simulink model "rovertest"  (R2023a)
settings: Solver=VariableStepAuto  StartTime=0.0  StopTime=60  RelTol=1e-3
libraries: robotalgslib x1
settings Model: Creator=ockap  LastModifiedBy=ockap

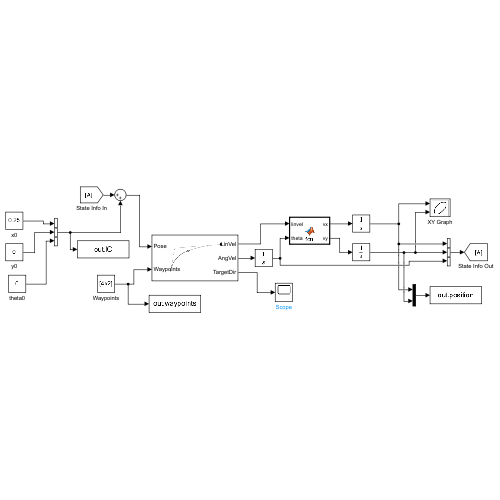
[thumbnail: Simulink's stored preview of the top-level diagram]
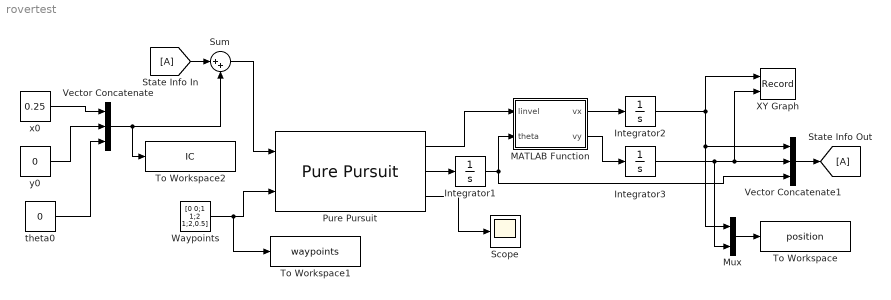
== system rovertest ==
  Integrator1 : Integrator
  Integrator2 : Integrator
  Integrator3 : Integrator
  MATLAB Function : MATLAB Function  TreatAsAtomicUnit=on
  Mux : Mux  Inputs=2
  Pure Pursuit : robotalgslib/Pure Pursuit  DesiredLinearVelocity=0.05  MaxAngularVelocity=1.0  LookaheadDistance=0.2  TargetDirPort=on  SimulateUsing=Code generation
      settings: LibrarySourceBlock=robotmobilelib/Pure Pursuit
  Scope : Scope
  State Info In : From
  State Info Out : Goto
  Sum : Sum  Inputs=|++
  To Workspace : ToWorkspace  VariableName=position  SaveFormat=Timeseries  SampleTime=-1
  To Workspace1 : ToWorkspace  VariableName=waypoints  SampleTime=-1
      settings: Save2DSignal=2-D array (concatenate along first dimension)
  To Workspace2 : ToWorkspace  VariableName=IC  SampleTime=-1
      settings: Save2DSignal=2-D array (concatenate along first dimension)
  Vector Concatenate : Concatenate  NumInputs=3
  Vector Concatenate1 : Concatenate  NumInputs=3
  Waypoints : Constant  Value=[0 0;1 1;2 1;2,0.5]  VectorParams1D=off
  XY Graph : Record  FileSettingsInternal="{\"entries\":[{\"content\":{\"excelSettings\":{\"content\":{},\"type\":\"Streamout.ExcelSettings\"}},\"type\":\"Streamout.FileSettingStorage\",\"uuid\":\"\"}],\"packageUris\":[\"http:\\/\\/schema.mathworks.com\\/mf0\\/streamout_blocks\\/R2020a\"],\"version\":\"1.0\"}"  Layout=[1 1]  SignalsInternal="{\"entries\":[{\"content\":{\"signals\":[{\"content\":{\"blockPath\":[],\"dimensions\":[1],\"domain\":\"\",\"lineColor\":\"#a2142f\",\"plots\":[1],\"port\":1,\"sid\":[\"\"],\"signalID\":19,\"signalName\":\"Integrator2\"},\"type\":\"RecordBlkView.Signal\",\"uuid\":\"\"},{\"content\":{\"blockPath\":[],\"dimensions\":[1],\"domain\":\"\",\"lineColor\":\"#139fff\",\"plots\":[1],\"port\":2,\"sid\":[\"\"],\"signalID\":23,\"signalName\":\"Integrator3\"},\"type\":\"RecordBlkView.Signal\",\"uuid\":\"\"}]},\"type\":\"RecordBlkView.InputSignals\",\"uuid\":\"\"}],\"packageUris\":[\"http:\\/\\/schema.mathworks.com\\/mf0\\/streamout_blocks\\/R2020a\"],\"version\":\"1.0\"}"  VisualizationBindings="{\"xyplotplugin\":{\"info\":[{\"series\":[{\"bindingParametersList\":[{\"parameter\":\"X-Axis\",\"signalID\":19,\"signalName\":\"Integrator2\"},{\"parameter\":\"Y-Axis\",\"signalID\":23,\"signalName\":\"Integrator3\"}],\"seriesID\":3777}],\"subplotID\":1}]}}"  CompatibilityTag=XY
  theta0 : Constant  Value=0
  x0 : Constant  Value=0.25
  y0 : Constant  Value=0
  wires:
  Pure Pursuit/2 -> Integrator1/1
  Pure Pursuit/3 -> Scope/1
  State Info In/1 -> Sum/1
  Pure Pursuit/1 -> MATLAB Function/1(linvel)
  Integrator1/1 -> Vector Concatenate1/3, MATLAB Function/2(theta)
  MATLAB Function/1(vx) -> Integrator2/1
  MATLAB Function/2(vy) -> Integrator3/1
  Integrator2/1 -> Mux/1, Vector Concatenate1/1, XY Graph/1
  Vector Concatenate1/1 -> State Info Out/1
  Sum/1 -> Pure Pursuit/1
  Vector Concatenate/1 -> To Workspace2/1, Sum/2
  x0/1 -> Vector Concatenate/1
  y0/1 -> Vector Concatenate/2
  theta0/1 -> Vector Concatenate/3
  Waypoints/1 -> To Workspace1/1, Pure Pursuit/2
  Integrator3/1 -> Vector Concatenate1/2, XY Graph/2, Mux/2
  Mux/1 -> To Workspace/1

== matlab function rovertest/MATLAB Function ==
  data: linvel input; vx output; theta input; vy output
function [vx,vy] = fcn(linvel,theta)
    vx = linvel*cos(theta);
    vy = linvel*sin(theta);
end
